simulink model "State_UA_Khoo_Borbely"  (Simulink 7.0)
settings: Solver=ode45  StartTime=0.0  StopTime=10.0  RelTol=1e-3
values from neighbouring files (symbols this model uses):
  Circadian_Period = 24    [Respiratory_IC.m]    (also in State_UA_Khoo_IC.m)
  fc = 0.4/60    (= 0.00666666666667)    [Respiratory_IC.m]    (also in State_UA_Khoo_IC.m)
  gc = 0.008/60    (= 0.000133333333333)    [Respiratory_IC.m]    (also in State_UA_Khoo_IC.m)
  R_CW = 1.03    [Pleural_Schuessler_IC.m]    (also in Pmus_Flow_Younes_IC.m; Resp_Mech_IC.m; Respiratory_IC.m)
  R_L = 1.69    [Pleural_Schuessler_IC.m]    (also in Pmus_Flow_Younes_IC.m; Resp_Mech_IC.m; Respiratory_IC.m)
  rc = 0.2/60    (= 0.00333333333333)    [Respiratory_IC.m]    (also in State_UA_Khoo_IC.m)
  SWAo = 0.007    [Respiratory_IC.m]    (also in State_UA_Khoo_IC.m)
  time_step = time_step    [acquire_data.m]    (also in acquire_data_save.m)
undefined symbols (not defined in the file or in its folder): A_0_ua, Arousal_UAIC, b_ua, C_ua_awake, DAY, K_ua, R_LAW, R_trachea
libraries: simulink x1, simulink_extras x1
settings Model: Creator=CLM  LastModifiedBy=CLM
settings OptimizationCC: BlockReduction=off  BooleanDataType=off
settings DebuggingCC: SaveWithParameterizedLinksMsg=none  SignalResolutionControl=TryResolveAllWithWarning  SolverPrmCheckMsg=none  MultiTaskDSMMsg=warning  MultiTaskCondExecSysMsg=none  StrictBusMsg=None
settings HardwareCC: TargetUnknown=on
settings RTWCC: IncludeERTFirstTime=on
settings GRTTargetCC: TargetFcnLib=ansi_tfl_tmw.mat

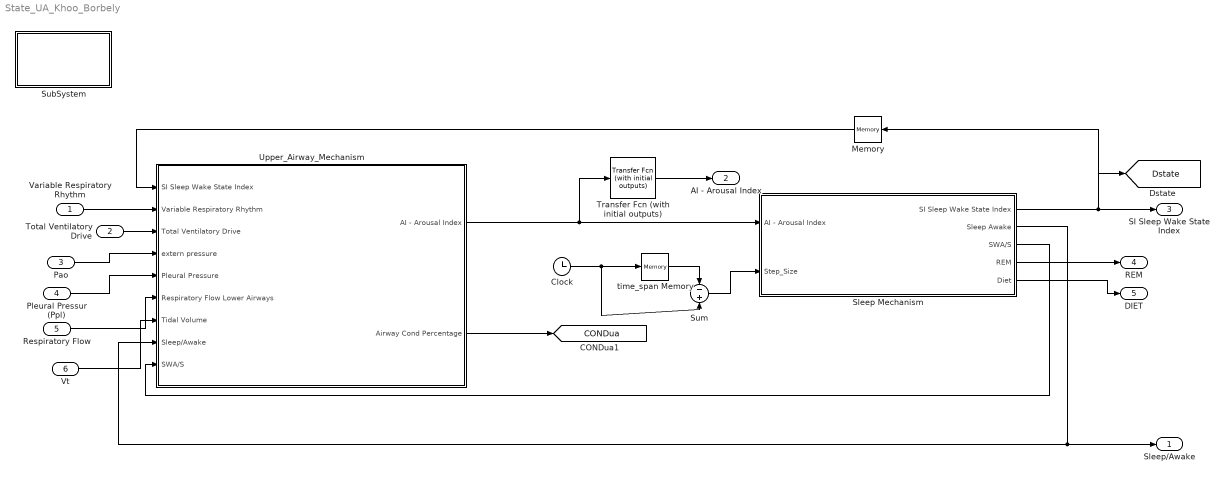
== system State_UA_Khoo_Borbely ==
  Variable Respiratory Rhythm : Inport  OutDataType=sfix(16)  OutScaling=2^0
  Total Ventilatory Drive : Inport  Port=2  OutDataType=sfix(16)  OutScaling=2^0
  Pao : Inport  Port=3  OutDataType=sfix(16)  OutScaling=2^0
  Pleural Pressur (Ppl) : Inport  Port=4  OutDataType=sfix(16)  OutScaling=2^0
  Respiratory Flow : Inport  Port=5  OutDataType=sfix(16)  OutScaling=2^0
  Vt : Inport  Port=6  OutDataType=sfix(16)  OutScaling=2^0
  Clock : Clock
      settings: Decimation=10
  Memory : Memory  Orientation=left  InheritSampleTime=on
  Sleep Mechanism : Subsystem
  SubSystem : Subsystem
      settings: OpenFcn=pneuma_variables
      mask Display: disp('"double click here"\n to load \nState_UA_Khoo \ninitial values');
  Sum : Sum  Inputs=-+  OutDataType=sfix(16)  OutScaling=2^0  SaturateOnIntegerOverflow=on  InputSameDT=on
  Transfer Fcn (with initial outputs) : simulink_extras/Additional Linear/Transfer Fcn (with initial outputs)  SystemSampleTime=-1  N=1  D=[5 1]  Y0=Arousal_CardIC  U0=Arousal_CardIC
  Upper_Airway_Mechanism : Subsystem
  time_span Memory : Memory  X0=0-time_step
  Sleep/Awake : Outport  OutDataType=sfix(16)  OutScaling=2^0
  AI - Arousal Index : Outport  Port=2  OutDataType=sfix(16)  OutScaling=2^0
  SI Sleep Wake State Index : Outport  Port=3  OutDataType=sfix(16)  OutScaling=2^0
  REM : Outport  Port=4  OutDataType=sfix(16)  OutScaling=2^0
  DIET : Outport  Port=5  OutDataType=sfix(16)  OutScaling=2^0
  tag scope: CONDua=global, Dstate=global
  wires:
  Total Ventilatory Drive/1 -> Upper_Airway_Mechanism/3(Total Ventilatory Drive)
  Upper_Airway_Mechanism/1(AI - Arousal Index) -> Sleep Mechanism/1(AI - Arousal Index), Transfer Fcn (with initial outputs)/1
  Memory/1 -> Upper_Airway_Mechanism/1(SI Sleep Wake State Index)
  Sleep Mechanism/1(SI Sleep Wake State Index) -> Memory/1, SI Sleep Wake State Index/1, [Dstate]
  Sleep Mechanism/2(Sleep Awake) -> Upper_Airway_Mechanism/8(Sleep/Awake), Sleep/Awake/1
  Upper_Airway_Mechanism/2("Airway Cond Percentage ") -> [CONDua]
  Variable Respiratory Rhythm/1 -> Upper_Airway_Mechanism/2(Variable Respiratory Rhythm)
  Sleep Mechanism/3(SWA/S) -> Upper_Airway_Mechanism/9(SWA/S)
  Transfer Fcn (with initial outputs)/1 -> AI - Arousal Index/1
  Sleep Mechanism/4(REM) -> REM/1
  Sleep Mechanism/5(Diet) -> DIET/1
  Pao/1 -> Upper_Airway_Mechanism/4(extern pressure)
  Pleural Pressur (Ppl)/1 -> Upper_Airway_Mechanism/5(Pleural Pressure)
  Respiratory Flow/1 -> Upper_Airway_Mechanism/6(Respiratory Flow Lower Airways)
  Vt/1 -> Upper_Airway_Mechanism/7(Tidal Volume)
  Clock/1 -> time_span Memory/1, Sum/2
  time_span Memory/1 -> Sum/1
  Sum/1 -> Sleep Mechanism/2(Step_Size)

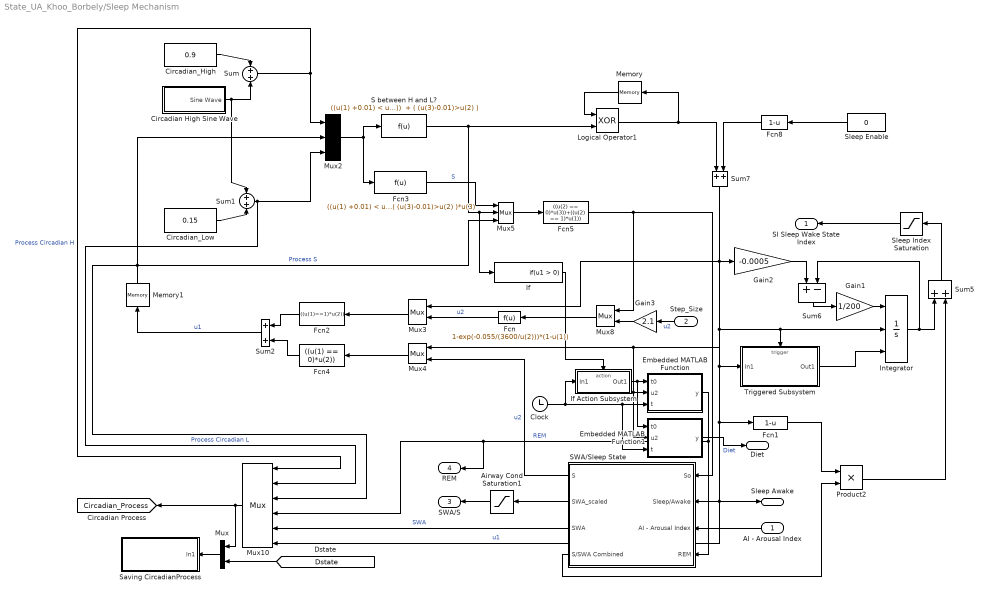
== system State_UA_Khoo_Borbely/Sleep Mechanism ==
  AI - Arousal Index : Inport  Orientation=left  OutDataType=sfix(16)  OutScaling=2^0
  Step_Size : Inport  Orientation=left  Port=2  OutDataType=sfix(16)  OutScaling=2^0
  Airway Cond Saturation1 : Saturate  Orientation=left  UpperLimit=1  LowerLimit=0
  Circadian High Sine Wave : Subsystem
  Circadian_High : Constant  Value=0.9  OutDataType=sfix(16)  OutScaling=2^0
  Circadian_Low : Constant  Value=0.15  OutDataType=sfix(16)  OutScaling=2^0
  Clock : Clock
      settings: Decimation=10
  Embedded MATLAB Function : Stateflow chart
  Embedded MATLAB Function1 : Stateflow chart
  Fcn : Fcn  Orientation=left  Expr=1-exp(-0.055/(3600/u(2)))*(1-u(1))
  Fcn1 : Fcn  Expr=1-u
  Fcn2 : Fcn  Orientation=left  Expr=((u(1)==1)*u(2))
  Fcn3 : Fcn  Expr=((u(1) +0.01) < u(2)) * u(1) + ( (u(3)-0.01)>u(2) )*u(3)
  Fcn4 : Fcn  Orientation=left  Expr=((u(1) == 0)*u(2))
  Fcn5 : Fcn  Expr=((u(2) == 0)*u(3))+((u(2) == 1)*u(1))
  Fcn8 : Fcn  Orientation=left  Expr=1-u
  Gain1 : Gain  Gain=1/200  ParameterDataType=sfix(16)  ParameterScaling=2^0  OutDataType=sfix(16)  OutScaling=2^0  SaturateOnIntegerOverflow=on
  Gain2 : Gain  Gain=-0.0005  ParameterDataType=sfix(16)  ParameterScaling=2^0  OutDataType=sfix(16)  OutScaling=2^0  SaturateOnIntegerOverflow=on
  Gain3 : Gain  Orientation=left  Gain=2.1  ParameterDataType=sfix(16)  ParameterScaling=2^0  OutDataType=sfix(16)  OutScaling=2^0  SaturateOnIntegerOverflow=on
  If : If  ShowElse=off
  If Action Subsystem : Subsystem  TreatAsAtomicUnit=on
  Integrator : Integrator  ExternalReset=rising  InitialConditionSource=external  InitialCondition=1
  Logical Operator1 : Logic  Operator=XOR
  Memory : Memory  Orientation=left  X0=1  InheritSampleTime=on
  Memory1 : Memory  Orientation=up  X0=1  InheritSampleTime=on
  Mux{,3..4,8} (4 alike) : Mux  Orientation=left  Inputs=2
  Mux10 : Mux  Orientation=left  Inputs=6
  Mux2 : Mux  Inputs=3
  Mux5 : Mux  Inputs=3
  Product2 : Product  OutDataType=sfix(16)  OutScaling=2^0  SaturateOnIntegerOverflow=on  InputSameDT=on
  S between H and L? : Fcn  Expr="((u(1) +0.01) < u(2))  + ( (u(3)-0.01)>u(2) )"
  SWA/Sleep State : Subsystem  Orientation=left
  Saving CircadianProcess : Subsystem  Orientation=left
  Sleep Enable : Constant  Orientation=left  Value=0  OutDataType=sfix(16)  OutScaling=2^0
  Sleep Index Saturation : Saturate  Orientation=left  UpperLimit=1  LowerLimit=0
  Sum : Sum  OutDataType=sfix(16)  OutScaling=2^0  SaturateOnIntegerOverflow=on  InputSameDT=on
  Sum1 : Sum  OutDataType=sfix(16)  OutScaling=2^0  SaturateOnIntegerOverflow=on  InputSameDT=on
  Sum2 : Sum  Orientation=left  OutDataType=sfix(16)  OutScaling=2^0  SaturateOnIntegerOverflow=on  InputSameDT=on
  Sum5 : Sum  Orientation=up  OutDataType=sfix(16)  OutScaling=2^0  SaturateOnIntegerOverflow=on  InputSameDT=on
  Sum6 : Sum  Orientation=down  Inputs=+-  OutDataType=sfix(16)  OutScaling=2^0  SaturateOnIntegerOverflow=on  InputSameDT=on
  Sum7 : Sum  Orientation=down  OutDataType=sfix(16)  OutScaling=2^0  SaturateOnIntegerOverflow=on  InputSameDT=on
  Triggered Subsystem : Subsystem  TreatAsAtomicUnit=on
  SI Sleep Wake State Index : Outport  Orientation=left  OutDataType=sfix(16)  OutScaling=2^0
  Sleep Awake : Outport  Port=2  OutDataType=sfix(16)  OutScaling=2^0
  SWA/S : Outport  Orientation=left  Port=3  OutDataType=sfix(16)  OutScaling=2^0
  REM : Outport  Orientation=left  Port=4  OutDataType=sfix(16)  OutScaling=2^0
  Diet : Outport  Port=5  OutDataType=sfix(16)  OutScaling=2^0
  tag scope: Circadian_Process=global
  wires:
  AI - Arousal Index/1 -> SWA/Sleep State/3(AI - Arousal Index)
  Circadian_High/1 -> Sum/1
  Circadian High Sine Wave/1(Sine Wave) -> Sum/2, Sum1/1
  Circadian_Low/1 -> Sum1/2
  Sum/1 -> Mux2/1, Mux10/1  "Process Circadian H"
  Sum1/1 -> Mux2/3, Mux10/2  "Process Circadian L"
  Memory/1 -> Logical Operator1/1
  Logical Operator1/1 -> Memory/1, Sum7/1
  Fcn3/1 -> Mux5/1  "S"
  Fcn2/1 -> Sum2/1
  Sum2/1 -> Memory1/1  "u1"
  Fcn/1 -> Mux3/2  "u2"
  SWA/Sleep State/1(S) -> Mux4/2  "u2"
  Mux5/1 -> Fcn5/1
  Mux3/1 -> Fcn2/1
  Mux4/1 -> Fcn4/1
  Fcn5/1 -> SWA/Sleep State/1(So), Mux8/1
  Mux8/1 -> Fcn/1
  Step_Size/1 -> Gain3/1  "u2"
  SWA/Sleep State/2(SWA_scaled) -> Airway Cond Saturation1/1
  Airway Cond Saturation1/1 -> SWA/S/1
  Mux10/1 -> [Circadian_Process], Mux/1
  SWA/Sleep State/3(SWA) -> Mux10/5  "SWA"
  SWA/Sleep State/4(S/SWA Combined) -> Product2/2
  Fcn1/1 -> Product2/1
  Sum5/1 -> Sleep Index Saturation/1
  Product2/1 -> Sum5/2
  Sleep Index Saturation/1 -> SI Sleep Wake State Index/1
  Sum7/1 -> Gain2/1, Mux3/1, Triggered Subsystem/Trigger, Integrator/2, Fcn1/1, Sleep Awake/1, SWA/Sleep State/2(Sleep/Awake), Mux10/6, Mux4/1, Embedded MATLAB Function/2(u2), Embedded MATLAB Function1/2(u2), Triggered Subsystem/1(In1)  "u1"
  Integrator/1 -> Sum5/1, Sum6/2
  Triggered Subsystem/1(Out1) -> Integrator/3
  Gain2/1 -> Sum6/1
  Sum6/1 -> Gain1/1
  Gain1/1 -> Integrator/1
  Fcn8/1 -> Sum7/2
  Memory1/1 -> Mux5/3, Mux10/3, Mux2/2  "Process S"
  Mux2/1 -> Fcn3/1, S between H and L?/1
  S between H and L?/1 -> Logical Operator1/2, Mux5/2, If/1
  Gain3/1 -> Mux8/2
  If Action Subsystem/1(Out1) -> Embedded MATLAB Function/1(t0), Embedded MATLAB Function1/1(t0)
  If/1 -> If Action Subsystem/Action
  Fcn4/1 -> Sum2/2
  Clock/1 -> If Action Subsystem/1(In1), Embedded MATLAB Function/3(t), Embedded MATLAB Function1/3(t)
  Embedded MATLAB Function/1(y) -> SWA/Sleep State/4(REM), Mux10/4, REM/1  "REM"
  Sleep Enable/1 -> Fcn8/1
  [Dstate] -> Mux/2
  Mux/1 -> Saving CircadianProcess/1(In1)
  Embedded MATLAB Function1/1(y) -> Diet/1  "Diet"

== system State_UA_Khoo_Borbely/SubSystem ==

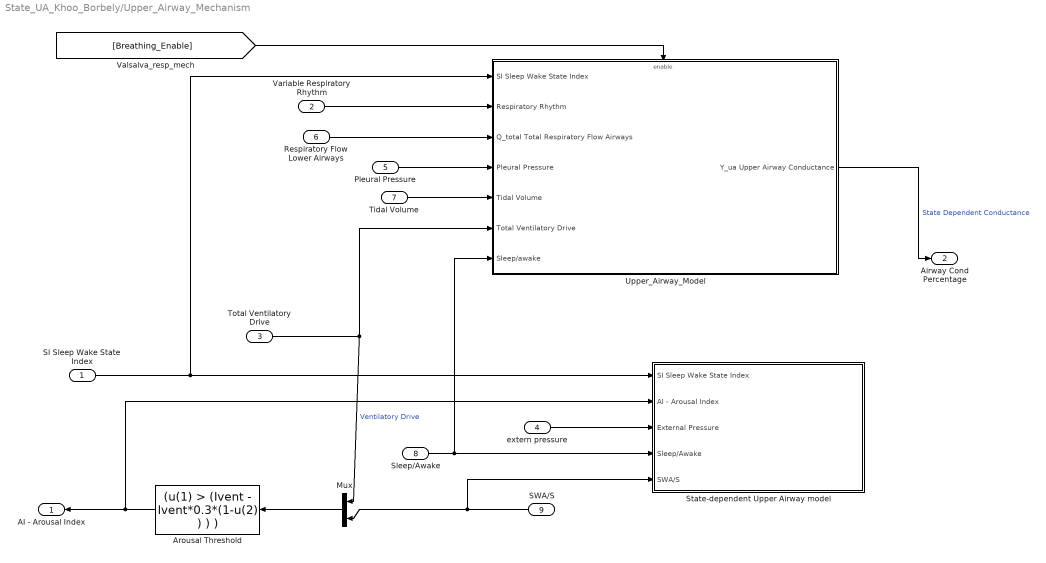
== system State_UA_Khoo_Borbely/Upper_Airway_Mechanism ==
  SI Sleep Wake State Index : Inport  OutDataType=sfix(16)  OutScaling=2^0
  Variable Respiratory Rhythm : Inport  Port=2  OutDataType=sfix(16)  OutScaling=2^0
  Total Ventilatory Drive : Inport  Port=3  OutDataType=sfix(16)  OutScaling=2^0
  extern pressure : Inport  Port=4  OutDataType=sfix(16)  OutScaling=2^0
  Pleural Pressure : Inport  Port=5  OutDataType=sfix(16)  OutScaling=2^0
  Respiratory Flow Lower Airways : Inport  Port=6  OutDataType=sfix(16)  OutScaling=2^0
  Tidal Volume : Inport  Port=7  OutDataType=sfix(16)  OutScaling=2^0
  Sleep/Awake : Inport  Port=8  OutDataType=sfix(16)  OutScaling=2^0
  SWA/S : Inport  Orientation=left  Port=9  OutDataType=sfix(16)  OutScaling=2^0
  Arousal Threshold : Fcn  Orientation=left  Expr=(u(1) > (Ivent - Ivent*0.3*(1-u(2) ) ) )
  Mux : Mux  Orientation=left  Inputs=2
  State-dependent Upper Airway model : Subsystem
  Upper_Airway_Model : Subsystem  TreatAsAtomicUnit=on
  AI - Arousal Index : Outport  Orientation=left  OutDataType=sfix(16)  OutScaling=2^0
  "Airway Cond Percentage " : Outport  Port=2  OutDataType=sfix(16)  OutScaling=2^0
  wires:
  SI Sleep Wake State Index/1 -> Upper_Airway_Model/1(SI Sleep Wake State Index), State-dependent Upper Airway model/1(SI Sleep Wake State Index)
  extern pressure/1 -> State-dependent Upper Airway model/3(External Pressure)
  SWA/S/1 -> Mux/2, State-dependent Upper Airway model/5(SWA/S)
  Total Ventilatory Drive/1 -> Upper_Airway_Model/6(Total Ventilatory Drive), Mux/1  "Ventilatory Drive"
  Sleep/Awake/1 -> State-dependent Upper Airway model/4(Sleep/Awake), Upper_Airway_Model/7(Sleep/awake)
  Upper_Airway_Model/1("Y_ua Upper Airway Conductance ") -> "Airway Cond Percentage "/1  "State Dependent Conductance"
  Variable Respiratory Rhythm/1 -> Upper_Airway_Model/2(Respiratory Rhythm)
  Respiratory Flow Lower Airways/1 -> Upper_Airway_Model/3(Q_total Total Respiratory Flow Airways)
  Pleural Pressure/1 -> Upper_Airway_Model/4(Pleural Pressure)
  Tidal Volume/1 -> Upper_Airway_Model/5(Tidal Volume)
  [Breathing_Enable] -> Upper_Airway_Model/Enable
  Mux/1 -> Arousal Threshold/1
  Arousal Threshold/1 -> AI - Arousal Index/1, State-dependent Upper Airway model/2(AI - Arousal Index)

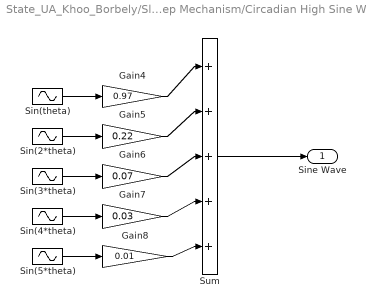
== system State_UA_Khoo_Borbely/Sleep Mechanism/Circadian High Sine Wave ==
  Gain4 : Gain  Gain=0.97  ParameterDataType=sfix(16)  ParameterScaling=2^0  OutDataType=sfix(16)  OutScaling=2^0  SaturateOnIntegerOverflow=on
  Gain5 : Gain  Gain=0.22  ParameterDataType=sfix(16)  ParameterScaling=2^0  OutDataType=sfix(16)  OutScaling=2^0  SaturateOnIntegerOverflow=on
  Gain6 : Gain  Gain=0.07  ParameterDataType=sfix(16)  ParameterScaling=2^0  OutDataType=sfix(16)  OutScaling=2^0  SaturateOnIntegerOverflow=on
  Gain7 : Gain  Gain=0.03  ParameterDataType=sfix(16)  ParameterScaling=2^0  OutDataType=sfix(16)  OutScaling=2^0  SaturateOnIntegerOverflow=on
  Gain8 : Gain  Gain=0.01  ParameterDataType=sfix(16)  ParameterScaling=2^0  OutDataType=sfix(16)  OutScaling=2^0  SaturateOnIntegerOverflow=on
  Sin(2*theta) : Sin  Amplitude=0.12  Frequency=0.00014544  Phase=3.2358  SampleTime=0
  Sin(3*theta) : Sin  Amplitude=0.12  Frequency=0.00021817  Phase=3.2358  SampleTime=0
  Sin(4*theta) : Sin  Amplitude=0.12  Frequency=0.00029089  Phase=3.2358  SampleTime=0
  Sin(5*theta) : Sin  Amplitude=0.12  Frequency=0.00036361  Phase=3.2358  SampleTime=0
  Sin(theta) : Sin  Amplitude=0.12  Frequency=7.2722e-005  Phase=3.2358  SampleTime=0
  Sum : Sum  Inputs=|+++++  OutDataType=sfix(16)  OutScaling=2^0  SaturateOnIntegerOverflow=on  InputSameDT=on
  Sine Wave : Outport  OutDataType=sfix(16)  OutScaling=2^0
  wires:
  Sin(theta)/1 -> Gain4/1
  Gain4/1 -> Sum/1
  Sin(2*theta)/1 -> Gain5/1
  Gain5/1 -> Sum/2
  Sin(3*theta)/1 -> Gain6/1
  Gain6/1 -> Sum/3
  Sin(4*theta)/1 -> Gain7/1
  Gain7/1 -> Sum/4
  Sin(5*theta)/1 -> Gain8/1
  Gain8/1 -> Sum/5
  Sum/1 -> Sine Wave/1

== system State_UA_Khoo_Borbely/Sleep Mechanism/If Action Subsystem ==
  In1 : Inport  OutDataType=sfix(16)  OutScaling=2^0
  Action Port : ActionPort
  Out1 : Outport  OutDataType=sfix(16)  OutScaling=2^0
  wires:
  In1/1 -> Out1/1

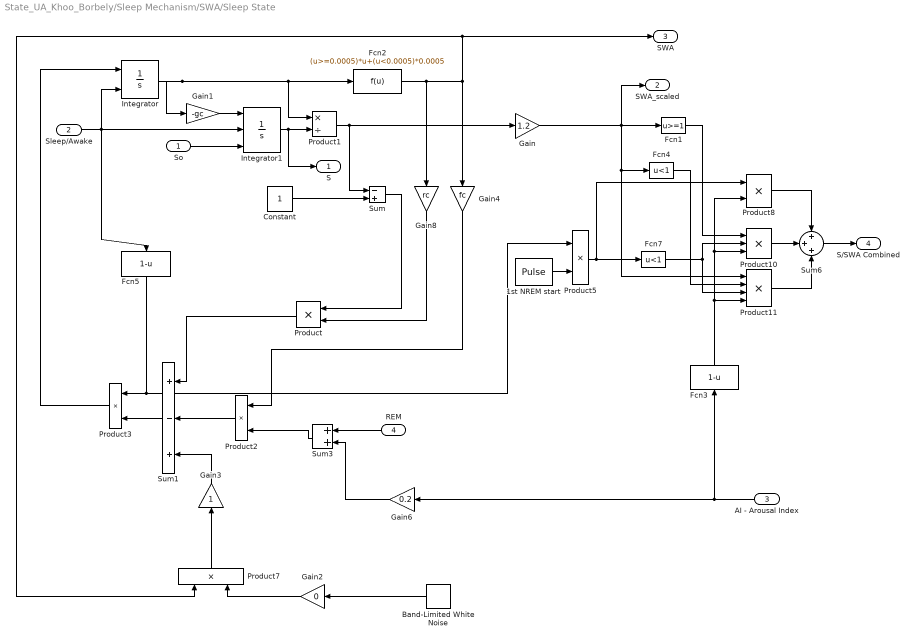
== system State_UA_Khoo_Borbely/Sleep Mechanism/SWA/Sleep State ==
  So : Inport  OutDataType=sfix(16)  OutScaling=2^0
  Sleep/Awake : Inport  Port=2  OutDataType=sfix(16)  OutScaling=2^0
  AI - Arousal Index : Inport  Orientation=left  Port=3  OutDataType=sfix(16)  OutScaling=2^0
  REM : Inport  Orientation=left  Port=4  OutDataType=sfix(16)  OutScaling=2^0
  1st NREM start : DiscretePulseGenerator  PulseType=Time based  Period=Circadian_Period*3600  PulseWidth=100 - 85 *1.8 /Circadian_Period  PhaseDelay=3600*1.8*0.85+5
  Band-Limited White Noise : simulink/Sources/Band-Limited White Noise  Orientation=left  SystemSampleTime=-1  Cov=[0.1]  Ts=0.1  seed=[23341]
  Constant : Constant  OutDataType=sfix(16)  OutScaling=2^0
  Fcn1 : Fcn  Expr=u>=1
  Fcn2 : Fcn  Expr=(u>=0.0005)*u+(u<0.0005)*0.0005
  Fcn3 : Fcn  Orientation=up  Expr=1-u
  Fcn4 : Fcn  Expr=u<1
  Fcn5 : Fcn  Orientation=down  Expr=1-u
  Fcn7 : Fcn  Expr=u<1
  Gain : Gain  Gain=1.2  ParameterDataType=sfix(16)  ParameterScaling=2^0  OutDataType=sfix(16)  OutScaling=2^0
  Gain1 : Gain  Gain=-gc  ParameterDataType=sfix(16)  ParameterScaling=2^0  OutDataType=sfix(16)  OutScaling=2^0  SaturateOnIntegerOverflow=on
  Gain2 : Gain  Orientation=left  Gain=0  ParameterDataType=sfix(16)  ParameterScaling=2^0  OutDataType=sfix(16)  OutScaling=2^0  SaturateOnIntegerOverflow=on
  Gain3 : Gain  Orientation=up  ParameterDataType=sfix(16)  ParameterScaling=2^0  OutDataType=sfix(16)  OutScaling=2^0  SaturateOnIntegerOverflow=on
  Gain4 : Gain  Orientation=down  Gain=fc  ParameterDataType=sfix(16)  ParameterScaling=2^0  OutDataType=sfix(16)  OutScaling=2^0  SaturateOnIntegerOverflow=on
  Gain6 : Gain  Orientation=left  Gain=0.2  ParameterDataType=sfix(16)  ParameterScaling=2^0  OutDataType=sfix(16)  OutScaling=2^0  SaturateOnIntegerOverflow=on
  Gain8 : Gain  Orientation=down  Gain=rc  ParameterDataType=sfix(16)  ParameterScaling=2^0  OutDataType=sfix(16)  OutScaling=2^0  SaturateOnIntegerOverflow=on
  Integrator : Integrator  ExternalReset=either  InitialCondition=SWAo  LimitOutput=on  UpperSaturationLimit=1  LowerSaturationLimit=0
  Integrator1 : Integrator  ExternalReset=falling  InitialConditionSource=external  InitialCondition=0.8  LimitOutput=on
  Product : Product  Orientation=left  OutDataType=sfix(16)  OutScaling=2^0  SaturateOnIntegerOverflow=on  InputSameDT=on
  Product1 : Product  Inputs=*/  OutDataType=sfix(16)  OutScaling=2^0  SaturateOnIntegerOverflow=on  InputSameDT=on
  Product10 : Product  Inputs=3  OutDataType=sfix(16)  OutScaling=2^0  SaturateOnIntegerOverflow=on  InputSameDT=on
  Product11 : Product  Inputs=4  OutDataType=sfix(16)  OutScaling=2^0  SaturateOnIntegerOverflow=on  InputSameDT=on
  Product2 : Product  Orientation=left  OutDataType=sfix(16)  OutScaling=2^0  SaturateOnIntegerOverflow=on  InputSameDT=on
  Product3 : Product  Orientation=left  OutDataType=sfix(16)  OutScaling=2^0  SaturateOnIntegerOverflow=on  InputSameDT=on
  Product5 : Product  Inputs=**  OutDataType=sfix(16)  OutScaling=2^0  SaturateOnIntegerOverflow=on  InputSameDT=on
  Product7 : Product  Orientation=up  OutDataType=sfix(16)  OutScaling=2^0  SaturateOnIntegerOverflow=on  InputSameDT=on
  Product8 : Product  OutDataType=sfix(16)  OutScaling=2^0  SaturateOnIntegerOverflow=on  InputSameDT=on
  Sum : Sum  Inputs=-+  OutDataType=sfix(16)  OutScaling=2^0  SaturateOnIntegerOverflow=on  InputSameDT=on
  Sum1 : Sum  Orientation=left  Inputs=+-+  OutDataType=sfix(16)  OutScaling=2^0  SaturateOnIntegerOverflow=on  InputSameDT=on
  Sum3 : Sum  Orientation=left  OutDataType=sfix(16)  OutScaling=2^0  SaturateOnIntegerOverflow=on  InputSameDT=on
  Sum6 : Sum  Inputs=+++  OutDataType=sfix(16)  OutScaling=2^0  SaturateOnIntegerOverflow=on  InputSameDT=on
  S : Outport  OutDataType=sfix(16)  OutScaling=2^0
  SWA_scaled : Outport  Port=2  OutDataType=sfix(16)  OutScaling=2^0
  SWA : Outport  Port=3  OutDataType=sfix(16)  OutScaling=2^0
  S/SWA Combined : Outport  Port=4  OutDataType=sfix(16)  OutScaling=2^0
  wires:
  Fcn4/1 -> Product11/2
  Fcn7/1 -> Product11/3, Product10/2
  Product10/1 -> Sum6/2
  Product11/1 -> Sum6/3
  Sum6/1 -> S/SWA Combined/1
  Product8/1 -> Sum6/1
  Gain2/1 -> Product7/2
  Product7/1 -> Gain3/1
  Gain6/1 -> Sum3/2
  AI - Arousal Index/1 -> Gain6/1, Fcn3/1
  Sum3/1 -> Product2/2
  Constant/1 -> Sum/2
  Product1/1 -> Sum/1, Gain/1
  Gain1/1 -> Integrator1/1
  Integrator/1 -> Product1/1, Fcn2/1, Gain1/1
  Sum/1 -> Product/1
  Product/1 -> Sum1/1
  Product2/1 -> Sum1/2
  Gain3/1 -> Sum1/3
  Integrator1/1 -> Product1/2, S/1
  Sleep/Awake/1 -> Integrator1/2, Fcn5/1, Integrator/2
  So/1 -> Integrator1/3
  Fcn2/1 -> Gain4/1, Product7/1, SWA/1, Gain8/1
  Gain/1 -> SWA_scaled/1, Fcn1/1, Product11/1, Fcn4/1
  Gain4/1 -> Product2/1
  Gain8/1 -> Product/2
  Sum1/1 -> Product3/2
  Product3/1 -> Integrator/1
  Fcn5/1 -> Product3/1, Product5/1
  Fcn3/1 -> Product8/2, Product10/3, Product11/4
  Band-Limited White Noise/1 -> Gain2/1
  Product5/1 -> Fcn7/1, Product8/1
  1st NREM start/1 -> Product5/2
  Fcn1/1 -> Product10/1
  REM/1 -> Sum3/1

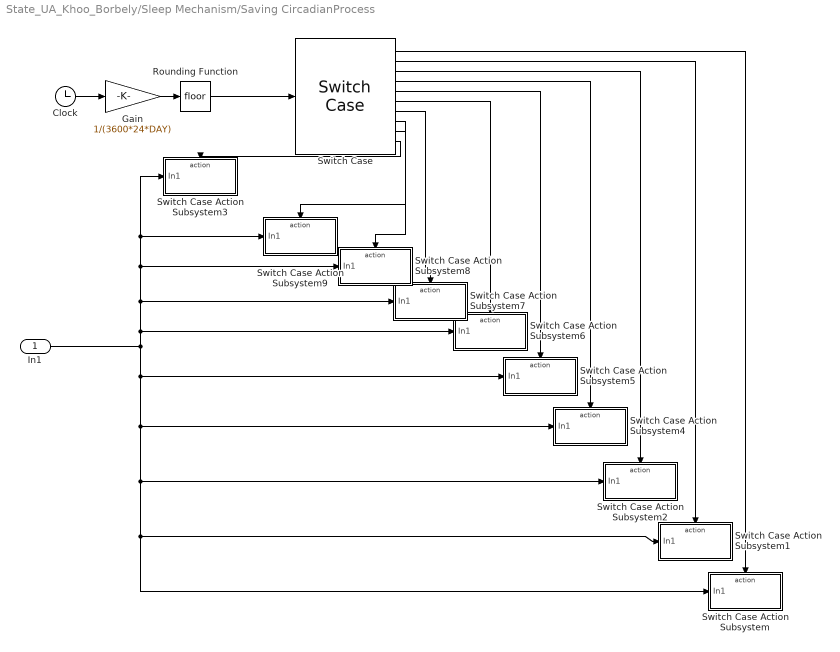
== system State_UA_Khoo_Borbely/Sleep Mechanism/Saving CircadianProcess ==
  In1 : Inport  OutDataType=sfix(16)  OutScaling=2^0
  Clock : Clock
      settings: Decimation=10
  Gain : Gain  Gain=1/(3600*24*DAY)  ParameterDataType=sfix(16)  ParameterScaling=2^0  OutDataType=sfix(16)  OutScaling=2^0
  Rounding Function : Rounding
  Switch Case : SwitchCase  CaseConditions={0,1,2,3,4,5,6,7,8}  SampleTime=sampletime
  Switch Case Action Subsystem : Subsystem  TreatAsAtomicUnit=on
  Switch Case Action Subsystem1 : Subsystem  TreatAsAtomicUnit=on
  Switch Case Action Subsystem2 : Subsystem  TreatAsAtomicUnit=on
  Switch Case Action Subsystem3 : Subsystem  TreatAsAtomicUnit=on
  Switch Case Action Subsystem4 : Subsystem  TreatAsAtomicUnit=on
  Switch Case Action Subsystem5 : Subsystem  TreatAsAtomicUnit=on
  Switch Case Action Subsystem6 : Subsystem  TreatAsAtomicUnit=on
  Switch Case Action Subsystem7 : Subsystem  TreatAsAtomicUnit=on
  Switch Case Action Subsystem8 : Subsystem  TreatAsAtomicUnit=on
  Switch Case Action Subsystem9 : Subsystem  TreatAsAtomicUnit=on
  wires:
  Clock/1 -> Gain/1
  Switch Case/1 -> Switch Case Action Subsystem/Action
  Switch Case/2 -> Switch Case Action Subsystem1/Action
  Switch Case/3 -> Switch Case Action Subsystem2/Action
  Switch Case/10 -> Switch Case Action Subsystem3/Action
  Rounding Function/1 -> Switch Case/1
  In1/1 -> Switch Case Action Subsystem/1(In1), Switch Case Action Subsystem1/1(In1), Switch Case Action Subsystem2/1(In1), Switch Case Action Subsystem5/1(In1), Switch Case Action Subsystem3/1(In1), Switch Case Action Subsystem9/1(In1), Switch Case Action Subsystem8/1(In1), Switch Case Action Subsystem7/1(In1), Switch Case Action Subsystem6/1(In1), Switch Case Action Subsystem4/1(In1)
  Gain/1 -> Rounding Function/1
  Switch Case/4 -> Switch Case Action Subsystem4/Action
  Switch Case/5 -> Switch Case Action Subsystem5/Action
  Switch Case/6 -> Switch Case Action Subsystem6/Action
  Switch Case/7 -> Switch Case Action Subsystem7/Action
  Switch Case/8 -> Switch Case Action Subsystem8/Action
  Switch Case/9 -> Switch Case Action Subsystem9/Action

== system State_UA_Khoo_Borbely/Sleep Mechanism/Triggered Subsystem ==
  In1 : Inport  OutDataType=sfix(16)  OutScaling=2^0
  Trigger : TriggerPort
  Out1 : Outport  OutDataType=sfix(16)  OutScaling=2^0
  wires:
  In1/1 -> Out1/1

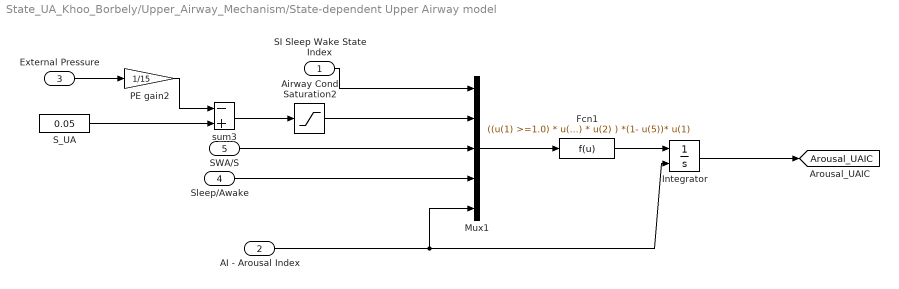
== system State_UA_Khoo_Borbely/Upper_Airway_Mechanism/State-dependent Upper Airway model ==
  SI Sleep Wake State Index : Inport  OutDataType=sfix(16)  OutScaling=2^0
  AI - Arousal Index : Inport  Port=2  OutDataType=sfix(16)  OutScaling=2^0
  External Pressure : Inport  Port=3  OutDataType=sfix(16)  OutScaling=2^0
  Sleep/Awake : Inport  Port=4  OutDataType=sfix(16)  OutScaling=2^0
  SWA/S : Inport  Port=5  OutDataType=sfix(16)  OutScaling=2^0
  Airway Cond Saturation2 : Saturate  UpperLimit=1  LowerLimit=0
  Fcn1 : Fcn  Expr="((u(1) >=1.0) * u(2) * (1 + 0.3 * (1 - u(3)) * (1-u(4)) )  + ( u(1)<1.0) * u(1) * u(2) ) *(1- u(5))* u(1)"
  Integrator : Integrator  ExternalReset=rising  InitialCondition=Arousal_UAIC
  Mux1 : Mux  Inputs=5
  PE gain2 : Gain  Gain=1/15  ParameterDataType=sfix(16)  ParameterScaling=2^0  OutDataType=sfix(16)  OutScaling=2^0  SaturateOnIntegerOverflow=on
  S_UA : Constant  Value=0.05  OutDataType=sfix(16)  OutScaling=2^0
  sum3 : Sum  Inputs=-+  OutDataType=sfix(16)  OutScaling=2^0  SaturateOnIntegerOverflow=on  InputSameDT=on
  tag scope: Arousal_UAIC=global
  wires:
  AI - Arousal Index/1 -> Integrator/2, Mux1/5
  SI Sleep Wake State Index/1 -> Mux1/1
  SWA/S/1 -> Mux1/3
  Sleep/Awake/1 -> Mux1/4
  S_UA/1 -> sum3/2
  sum3/1 -> Airway Cond Saturation2/1
  External Pressure/1 -> PE gain2/1
  PE gain2/1 -> sum3/1
  Mux1/1 -> Fcn1/1
  Airway Cond Saturation2/1 -> Mux1/2
  Fcn1/1 -> Integrator/1
  Integrator/1 -> [Arousal_UAIC]

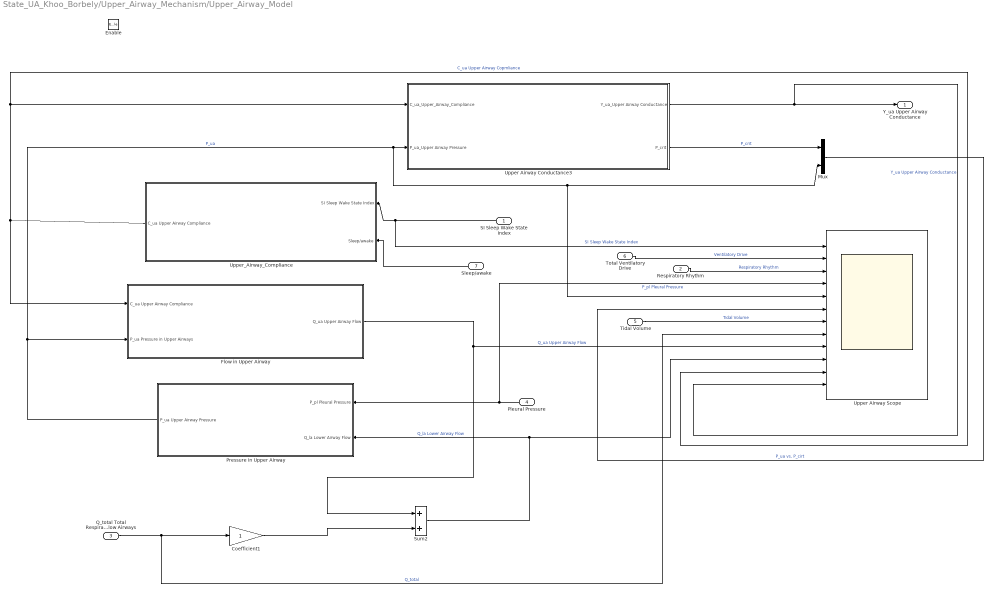
== system State_UA_Khoo_Borbely/Upper_Airway_Mechanism/Upper_Airway_Model ==
  SI Sleep Wake State Index : Inport  Orientation=left  OutDataType=sfix(16)  OutScaling=2^0
  Respiratory Rhythm : Inport  Port=2  OutDataType=sfix(16)  OutScaling=2^0
  Q_total Total Respiratory Flow Airways : Inport  Port=3  OutDataType=sfix(16)  OutScaling=2^0
  Pleural Pressure : Inport  Orientation=left  Port=4  OutDataType=sfix(16)  OutScaling=2^0
  Tidal Volume : Inport  Port=5  OutDataType=sfix(16)  OutScaling=2^0
  Total Ventilatory Drive : Inport  Port=6  OutDataType=sfix(16)  OutScaling=2^0
  Sleep/awake : Inport  Orientation=left  Port=7  OutDataType=sfix(16)  OutScaling=2^0
  Enable : EnablePort
  " Flow in Upper Airway" : Subsystem
  " Pressure in Upper Airway" : Subsystem  Orientation=left
  Coefficient1 : Gain  ParameterDataType=sfix(16)  ParameterScaling=2^0  OutDataType=sfix(16)  OutScaling=2^0  SaturateOnIntegerOverflow=on
  Mux : Mux  Inputs=2
  Sum2 : Sum  OutDataType=sfix(16)  OutScaling=2^0  SaturateOnIntegerOverflow=on
  Upper Airway Conductance3 : Subsystem
  Upper Airway Scope : Scope  NumInputPorts=12
      settings: TimeRange=120  YMin=0~0.2~-0.05~-40~-4~-41~-0.1~-2~-2e-006~-4~0.005~0.5  YMax=1~0.48~1.05~5~1.5~10~3~2.5~5e-006~5~0.01~1.05  SaveName=ScopeData20  MaxDataPoints=50
  Upper_Airway_Compliance : Subsystem  Orientation=left
  "Y_ua Upper Airway Conductance " : Outport  OutDataType=sfix(16)  OutScaling=2^0  InitialOutput=[0]
  wires:
  Q_total Total Respiratory Flow Airways/1 -> Upper Airway Scope/8, Coefficient1/1  "Q_total"
  SI Sleep Wake State Index/1 -> Upper_Airway_Compliance/1("SI Sleep Wake State Index "), Upper Airway Scope/1  "SI Sleep Wake State Index"
  Pleural Pressure/1 -> Upper Airway Scope/4, " Pressure in Upper Airway"/1(P_pl Pleural Pressure)  "P_pl Pleural Pressure"
  Sum2/1 -> " Pressure in Upper Airway"/2(Q_la Lower Airway Flow), Upper Airway Scope/10  "Q_la Lower Airway Flow"
  " Pressure in Upper Airway"/1("P_ua Upper Airway Pressure ") -> " Flow in Upper Airway"/2(P_ua Pressure in Upper Airways), Upper Airway Conductance3/2(P_ua_Upper Airway Pressure), Mux/2, Upper Airway Scope/5  "P_ua"
  Upper Airway Conductance3/2(P_crit) -> Mux/1  "P_crit"
  Upper_Airway_Compliance/1(C_ua Upper Airway Compliance) -> " Flow in Upper Airway"/1(C_ua Upper Airway Compliance), Upper Airway Conductance3/1(C_ua_Upper_Airway_Compliance), Upper Airway Scope/11  "C_ua Upper Airway Copmliance"
  " Flow in Upper Airway"/1("Q_ua Upper Airway Flow ") -> Upper Airway Scope/9, Sum2/1  "Q_ua Upper Airway Flow"
  Upper Airway Conductance3/1(Y_ua_Upper Airway Conductance) -> Upper Airway Scope/12, "Y_ua Upper Airway Conductance "/1  "Y_ua Upper Airway Conductance"
  Total Ventilatory Drive/1 -> Upper Airway Scope/2  "Ventilatory Drive"
  Mux/1 -> Upper Airway Scope/6  "P_ua vs. P_cirt"
  Tidal Volume/1 -> Upper Airway Scope/7  "Tidal Volume"
  Respiratory Rhythm/1 -> Upper Airway Scope/3  "Respiratory Rhythm"
  Sleep/awake/1 -> Upper_Airway_Compliance/2(Sleep/awake)
  Coefficient1/1 -> Sum2/2

== system State_UA_Khoo_Borbely/Sleep Mechanism/Saving CircadianProcess/Switch Case Action Subsystem ==
  In1 : Inport  OutDataType=sfix(16)  OutScaling=2^0
  Action Port : ActionPort
  To File : ToFile  Filename=CircadianProcess1.mat  MatrixName=H_L_CircardianLow_RBM_SWA  SampleTime=sampletime
  wires:
  In1/1 -> To File/1

== system State_UA_Khoo_Borbely/Sleep Mechanism/Saving CircadianProcess/Switch Case Action Subsystem1 ==
  In1 : Inport  OutDataType=sfix(16)  OutScaling=2^0
  Action Port : ActionPort
  To File : ToFile  Filename=CircadianProcess2.mat  MatrixName=H_L_CircardianLow_RBM_SWA  SampleTime=sampletime
  wires:
  In1/1 -> To File/1

== system State_UA_Khoo_Borbely/Sleep Mechanism/Saving CircadianProcess/Switch Case Action Subsystem2 ==
  In1 : Inport  OutDataType=sfix(16)  OutScaling=2^0
  Action Port : ActionPort
  To File : ToFile  Filename=CircadianProcess3.mat  MatrixName=H_L_CircardianLow_RBM_SWA  SampleTime=sampletime
  wires:
  In1/1 -> To File/1

== system State_UA_Khoo_Borbely/Sleep Mechanism/Saving CircadianProcess/Switch Case Action Subsystem3 ==
  In1 : Inport  OutDataType=sfix(16)  OutScaling=2^0
  Action Port : ActionPort
  To File : ToFile  Filename=CircadianProcess10.mat  MatrixName=H_L_CircardianLow_RBM_SWA  SampleTime=sampletime
  wires:
  In1/1 -> To File/1

== system State_UA_Khoo_Borbely/Sleep Mechanism/Saving CircadianProcess/Switch Case Action Subsystem4 ==
  In1 : Inport  OutDataType=sfix(16)  OutScaling=2^0
  Action Port : ActionPort
  To File : ToFile  Filename=CircadianProcess4.mat  MatrixName=H_L_CircardianLow_RBM_SWA  SampleTime=sampletime
  wires:
  In1/1 -> To File/1

== system State_UA_Khoo_Borbely/Sleep Mechanism/Saving CircadianProcess/Switch Case Action Subsystem5 ==
  In1 : Inport  OutDataType=sfix(16)  OutScaling=2^0
  Action Port : ActionPort
  To File : ToFile  Filename=CircadianProcess5.mat  MatrixName=H_L_CircardianLow_RBM_SWA  SampleTime=sampletime
  wires:
  In1/1 -> To File/1

== system State_UA_Khoo_Borbely/Sleep Mechanism/Saving CircadianProcess/Switch Case Action Subsystem6 ==
  In1 : Inport  OutDataType=sfix(16)  OutScaling=2^0
  Action Port : ActionPort
  To File : ToFile  Filename=CircadianProcess6.mat  MatrixName=H_L_CircardianLow_RBM_SWA  SampleTime=sampletime
  wires:
  In1/1 -> To File/1

== system State_UA_Khoo_Borbely/Sleep Mechanism/Saving CircadianProcess/Switch Case Action Subsystem7 ==
  In1 : Inport  OutDataType=sfix(16)  OutScaling=2^0
  Action Port : ActionPort
  To File : ToFile  Filename=CircadianProcess7.mat  MatrixName=H_L_CircardianLow_RBM_SWA  SampleTime=sampletime
  wires:
  In1/1 -> To File/1

== system State_UA_Khoo_Borbely/Sleep Mechanism/Saving CircadianProcess/Switch Case Action Subsystem8 ==
  In1 : Inport  OutDataType=sfix(16)  OutScaling=2^0
  Action Port : ActionPort
  To File : ToFile  Filename=CircadianProcess8.mat  MatrixName=H_L_CircardianLow_RBM_SWA  SampleTime=sampletime
  wires:
  In1/1 -> To File/1

== system State_UA_Khoo_Borbely/Sleep Mechanism/Saving CircadianProcess/Switch Case Action Subsystem9 ==
  In1 : Inport  OutDataType=sfix(16)  OutScaling=2^0
  Action Port : ActionPort
  To File : ToFile  Filename=CircadianProcess9.mat  MatrixName=H_L_CircardianLow_RBM_SWA  SampleTime=sampletime
  wires:
  In1/1 -> To File/1

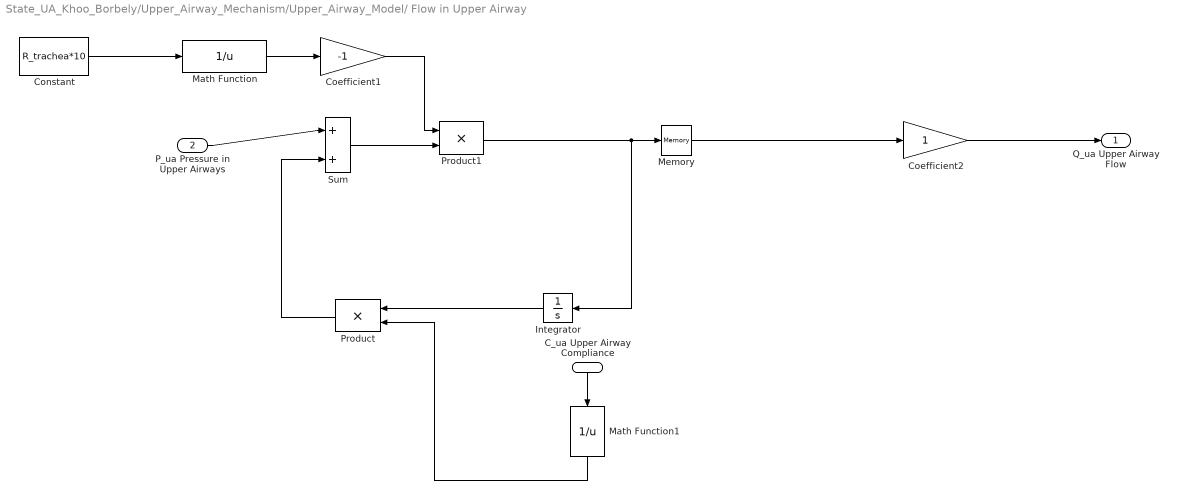
== system State_UA_Khoo_Borbely/Upper_Airway_Mechanism/Upper_Airway_Model/ Flow in Upper Airway ==
  C_ua Upper Airway Compliance : Inport  Orientation=down  OutDataType=sfix(16)  OutScaling=2^0
  P_ua Pressure in Upper Airways : Inport  Port=2  OutDataType=sfix(16)  OutScaling=2^0
  Coefficient1 : Gain  Gain=-1  ParameterDataType=sfix(16)  ParameterScaling=2^0  OutDataType=sfix(16)  OutScaling=2^0  SaturateOnIntegerOverflow=on
  Coefficient2 : Gain  ParameterDataType=sfix(16)  ParameterScaling=2^0  OutDataType=sfix(16)  OutScaling=2^0  SaturateOnIntegerOverflow=on
  Constant : Constant  Value=R_trachea*10  OutDataType=sfix(16)  OutScaling=2^0
  Integrator : Integrator  Orientation=left  LimitOutput=on  UpperSaturationLimit=100  LowerSaturationLimit=-100
  Math Function : Math  Operator=reciprocal  OutDataType=sfix(16)  OutScaling=2^0  SaturateOnIntegerOverflow=on
  Math Function1 : Math  Orientation=down  Operator=reciprocal  OutDataType=sfix(16)  OutScaling=2^0  SaturateOnIntegerOverflow=on
  Memory : Memory
  Product : Product  Orientation=left  OutDataType=sfix(16)  OutScaling=2^0  SaturateOnIntegerOverflow=on
  Product1 : Product  OutDataType=sfix(16)  OutScaling=2^0  SaturateOnIntegerOverflow=on
  Sum : Sum  Inputs=|++  OutDataType=sfix(16)  OutScaling=2^0  SaturateOnIntegerOverflow=on
  "Q_ua Upper Airway Flow " : Outport  OutDataType=sfix(16)  OutScaling=2^0
  wires:
  Product1/1 -> Integrator/1, Memory/1
  P_ua Pressure in Upper Airways/1 -> Sum/1
  Sum/1 -> Product1/2
  C_ua Upper Airway Compliance/1 -> Math Function1/1
  Integrator/1 -> Product/1
  Product/1 -> Sum/2
  Constant/1 -> Math Function/1
  Math Function/1 -> Coefficient1/1
  Coefficient1/1 -> Product1/1
  Coefficient2/1 -> "Q_ua Upper Airway Flow "/1
  Memory/1 -> Coefficient2/1
  Math Function1/1 -> Product/2

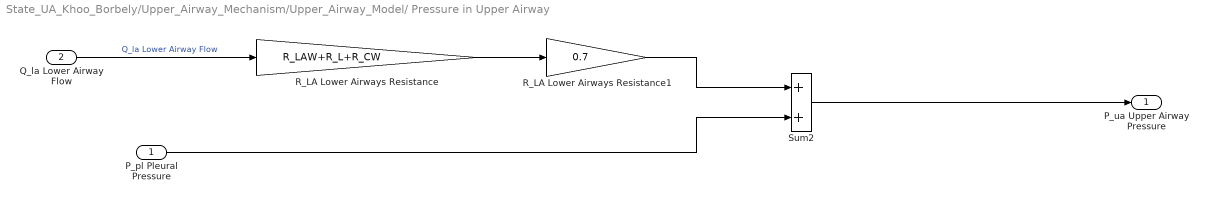
== system State_UA_Khoo_Borbely/Upper_Airway_Mechanism/Upper_Airway_Model/ Pressure in Upper Airway ==
  P_pl Pleural Pressure : Inport  OutDataType=sfix(16)  OutScaling=2^0
  Q_la Lower Airway Flow : Inport  Port=2  OutDataType=sfix(16)  OutScaling=2^0
  R_LA Lower Airways Resistance : Gain  Gain=R_LAW+R_L+R_CW  ParameterDataType=sfix(16)  ParameterScaling=2^0  OutDataType=sfix(16)  OutScaling=2^0  SaturateOnIntegerOverflow=on
  R_LA Lower Airways Resistance1 : Gain  Gain=0.7  ParameterDataType=sfix(16)  ParameterScaling=2^0  OutDataType=sfix(16)  OutScaling=2^0  SaturateOnIntegerOverflow=on
  Sum2 : Sum  OutDataType=sfix(16)  OutScaling=2^0  SaturateOnIntegerOverflow=on
  "P_ua Upper Airway Pressure " : Outport  OutDataType=sfix(16)  OutScaling=2^0  InitialOutput=[0]
  wires:
  Q_la Lower Airway Flow/1 -> R_LA Lower Airways Resistance/1  "Q_la Lower Airway Flow"
  P_pl Pleural Pressure/1 -> Sum2/2
  Sum2/1 -> "P_ua Upper Airway Pressure "/1
  R_LA Lower Airways Resistance/1 -> R_LA Lower Airways Resistance1/1
  R_LA Lower Airways Resistance1/1 -> Sum2/1

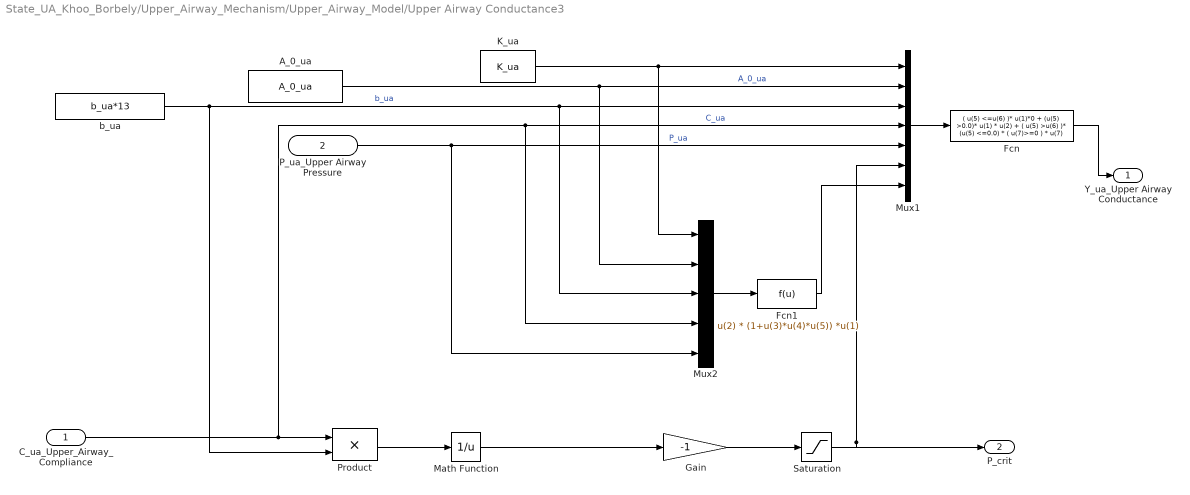
== system State_UA_Khoo_Borbely/Upper_Airway_Mechanism/Upper_Airway_Model/Upper Airway Conductance3 ==
  C_ua_Upper_Airway_Compliance : Inport  OutDataType=sfix(16)  OutScaling=2^0
  P_ua_Upper Airway Pressure : Inport  Port=2  OutDataType=sfix(16)  OutScaling=2^0
  A_0_ua : Constant  Value=A_0_ua  OutDataType=sfix(16)  OutScaling=2^0
  Fcn : Fcn  Expr="( u(5) <=u(6) )* u(1)*0  + (u(5) >0.0)* u(1) * u(2) +  ( u(5) >u(6) )* (u(5) <=0.0) * ( u(7)>=0 ) * u(7)"
  Fcn1 : Fcn  Expr=u(2) * (1+u(3)*u(4)*u(5)) *u(1)
  Gain : Gain  Gain=-1  ParameterDataType=sfix(16)  ParameterScaling=2^0  OutDataType=sfix(16)  OutScaling=2^0  SaturateOnIntegerOverflow=on
  K_ua : Constant  Value=K_ua  OutDataType=sfix(16)  OutScaling=2^0
  Math Function : Math  Operator=reciprocal  OutDataType=sfix(16)  OutScaling=2^0  SaturateOnIntegerOverflow=on
  Mux1 : Mux  Inputs=7
  Mux2 : Mux  Inputs=5
  Product : Product  OutDataType=sfix(16)  OutScaling=2^0  SaturateOnIntegerOverflow=on
  Saturation : Saturate  UpperLimit=10  LowerLimit=-40
  b_ua : Constant  Value=b_ua*13  OutDataType=sfix(16)  OutScaling=2^0
  Y_ua_Upper Airway Conductance : Outport  OutDataType=sfix(16)  OutScaling=2^0
  P_crit : Outport  Port=2  OutDataType=sfix(16)  OutScaling=2^0
  wires:
  P_ua_Upper Airway Pressure/1 -> Mux1/5, Mux2/5  "P_ua"
  K_ua/1 -> Mux1/1, Mux2/1
  C_ua_Upper_Airway_Compliance/1 -> Mux1/4, Mux2/4, Product/1  "C_ua"
  b_ua/1 -> Mux1/3, Mux2/3, Product/2  "b_ua"
  A_0_ua/1 -> Mux1/2, Mux2/2  "A_0_ua"
  Mux1/1 -> Fcn/1
  Fcn/1 -> Y_ua_Upper Airway Conductance/1
  Fcn1/1 -> Mux1/7
  Mux2/1 -> Fcn1/1
  Gain/1 -> Saturation/1
  Product/1 -> Math Function/1
  Math Function/1 -> Gain/1
  Saturation/1 -> P_crit/1, Mux1/6

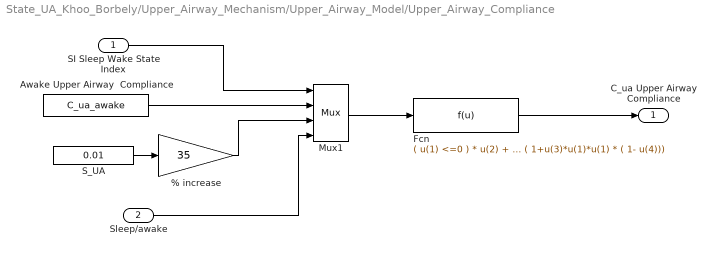
== system State_UA_Khoo_Borbely/Upper_Airway_Mechanism/Upper_Airway_Model/Upper_Airway_Compliance ==
  "SI Sleep Wake State Index " : Inport  OutDataType=sfix(16)  OutScaling=2^0
  Sleep/awake : Inport  Port=2  OutDataType=sfix(16)  OutScaling=2^0
  % increase : Gain  Gain=35  ParameterDataType=sfix(16)  ParameterScaling=2^0  OutDataType=sfix(16)  OutScaling=2^0  SaturateOnIntegerOverflow=on
  Awake Upper Airway  Compliance : Constant  Value=C_ua_awake  OutDataType=sfix(16)  OutScaling=2^0
  Fcn : Fcn  Expr="( u(1) <=0 ) * u(2) + ( u(1) >=1) * u(2) * ( 1+u(3) ) +  ( u(1) >0 ) * ( u(1) <1 ) * u(2) * ( 1+u(3)*u(1)*u(1) * ( 1- u(4)))"
  Mux1 : Mux
  S_UA : Constant  Value=0.01  OutDataType=sfix(16)  OutScaling=2^0
  C_ua Upper Airway Compliance : Outport  OutDataType=sfix(16)  OutScaling=2^0
  wires:
  Awake Upper Airway  Compliance/1 -> Mux1/2
  "SI Sleep Wake State Index "/1 -> Mux1/1
  % increase/1 -> Mux1/3
  Mux1/1 -> Fcn/1
  Fcn/1 -> C_ua Upper Airway Compliance/1
  S_UA/1 -> % increase/1
  Sleep/awake/1 -> Mux1/4

== matlab function Sleep Mechanism/Embedded MATLAB Function1 ==
  data: t0 input inherited; u2 input inherited; y output inherited; t input inherited
function y = fcn(t0, u2, t)
% This block supports an embeddable subset of the MATLAB language.
% See the help menu for details. 

% day = floor(para/3600/24);
% t0 = 0;
% count = 0;
% while count <=day
% if u1>0.5 %sleep/awake state change
%     t0 = t
% end
if u2 <0.5 %sleep start %sleep/awake state change
    y=0;
else %u2 >0.5 %(awake state)
    if (t>= t0 + 0.5*3600+5) && (t <= t0 + 0.5*3600+15*60+5)   %Breakfast
        y=22/60;
    elseif (t>= t0 + 5.5*3600+5) && (t <= t0 + 5.5*3600+30*60+5)%Lunch
        y=30/60;
    elseif (t>= t0 + 12*3600+5) && (t <=t0 + 12*3600+45*60+5)%dinner
        y=24/60;
    else %NREMs
        y=0; 
    end

end

== matlab function Sleep Mechanism/Embedded MATLAB Function ==
  data: t0 input inherited; u2 input inherited; y output inherited; t input inherited
function y = fcn(t0, u2, t)
% This block supports an embeddable subset of the MATLAB language.
% See the help menu for details. 

% day = floor(para/3600/24);
% t0 = 0;
% count = 0;
% while count <=day
% if u1>0.5 %sleep/awake state change
%     t0 = t
% end
if u2 >0.5 %awake state %sleep/awake state change
    y=0;
else %u2 <0.5 %(sleep start)
    if (t>=t0 + 0.85*1.8*3600+5) && (t <=t0 + 1*1.8*3600+5)   %1st REM
        y=1;
    elseif (t>=t0 + (1+0.85)*1.8*3600+5) && (t <=t0 + 2*1.8*3600+5)%2nd REM
        y=1;
    elseif (t>=t0 + (2+0.85)*1.8*3600+5) && (t <=t0 + 3*1.8*3600+5)%3rd REM
        y=1;
    elseif (t>=t0 + (3+0.85)*1.8*3600+5) && (t <=t0 + 4*1.8*3600+5)%4 REM
        y=1;
    elseif (t>=t0 + (4+0.85)*1.8*3600+5) && (t <=t0 + 5*1.8*3600+5)%5 REM
        y=1;
    elseif (t>=t0 + (5+0.85)*1.8*3600+5) && (t <=t0 + 6*1.8*3600+5)%6 REM
        y=1;
    else %NREMs
        y=0; 
    end

end
